simulink model "pseudo_calibrate"  (R2020b)
settings: Solver=VariableStepAuto  StartTime=0.0  StopTime=10  RelTol=1e-3
values from neighbouring files (symbols this model uses):
  B = 0.05    [md.m]    (also in pid.m; pinolo.m)
  J = 0.008    [md.m]    (also in pid.m; pinolo.m)
  KM = 0.22    [md.m]    (also in pid.m; pinolo.m)
  L = 0.0014    [md.m]    (also in pid.m; pinolo.m)
  MAX_SPEED = 330    [md.m]    (also in pid.m; pinolo.m)
  R = 2    [md.m]    (also in pid.m; pinolo.m)
  th = 50    [md.m]    (also in pid.m; pinolo.m)
  tl = 40    [md.m]    (also in pid.m; pinolo.m)
undefined symbols (not defined in the file or in its folder): den, num
libraries: simulink x2
settings Model: Creator=Titania  LastModifiedBy=Titania

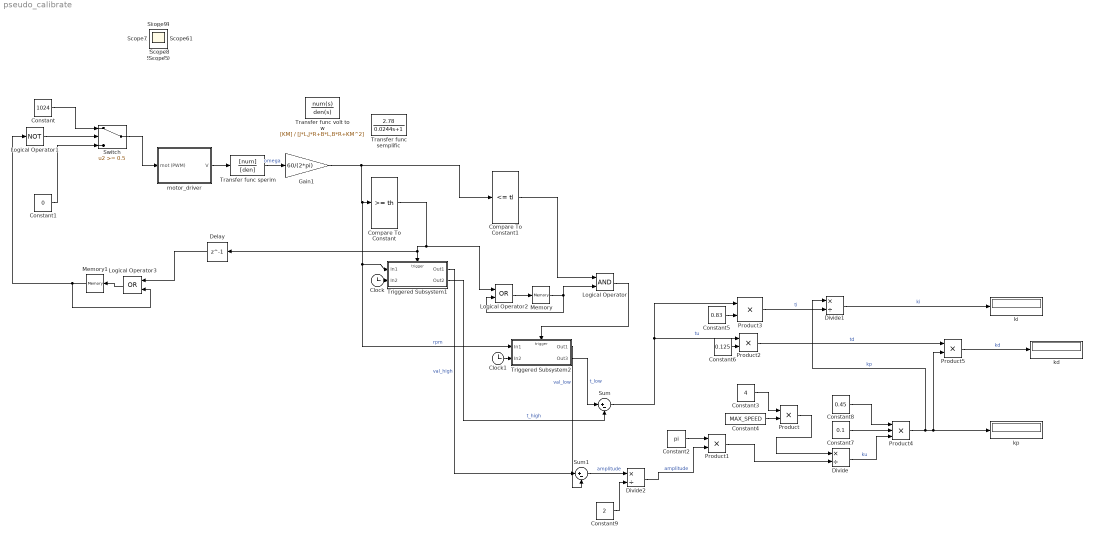
== system pseudo_calibrate ==
  Clock : Clock
  Clock1 : Clock
  Compare To Constant : simulink/Logic and Bit Operations/Compare To Constant  relop=>=  const=th  OutDataTypeStr=boolean
  Compare To Constant1 : simulink/Logic and Bit Operations/Compare To Constant  relop=<=  const=tl  OutDataTypeStr=boolean
  Constant : Constant  Value=1024
  Constant1 : Constant  Value=0
  Constant2 : Constant  Value=pi
  Constant3 : Constant  Value=4
  Constant4 : Constant  Value=MAX_SPEED
  Constant5 : Constant  Value=0.83
  Constant6 : Constant  Value=0.125
  Constant7 : Constant  Value=0.1
  Constant8 : Constant  Value=0.45
  Constant9 : Constant  Value=2
  Delay : Delay  DelayLength=1  InitialCondition=0
  Divide : Product  Inputs=*/
  Divide1 : Product  Inputs=*/
  Divide2 : Product  Inputs=*/
  Gain1 : Gain  Gain=60/(2*pi)
  Logical Operator : Logic  AllPortsSameDT=off  OutDataTypeStr=boolean
  Logical Operator1 : Logic  Operator=NOT  AllPortsSameDT=off  OutDataTypeStr=boolean
  Logical Operator2 : Logic  Operator=OR  AllPortsSameDT=off  OutDataTypeStr=boolean
  Logical Operator3 : Logic  Operator=OR  AllPortsSameDT=off  OutDataTypeStr=boolean
  Memory : Memory
  Memory1 : Memory
  Product{,1..3,5} (5 alike) : Product
  Product4 : Product  Inputs=3  OutDataTypeStr=single
  Sum : Sum  Inputs=|+-
  Sum1 : Sum  Inputs=|+-
  Switch : Switch  Threshold=0.5
  Transfer func semplific : TransferFcn  Numerator=[2.78]  Denominator=[0.0244,1]
  Transfer func sperim : TransferFcn  Numerator=[num]  Denominator=[den]
  Transfer func volt to w : TransferFcn  Numerator=[KM]  Denominator=[J*L,J*R+B*L,B*R+KM^2]
  Triggered Subsystem1 : Subsystem  TreatAsAtomicUnit=on
  Triggered Subsystem2 : Subsystem  TreatAsAtomicUnit=on
  kd : Display
  ki : Display
  kp : Display
  motor_driver : Subsystem
  Scope{,1..11} (12 alike) : Scope
  wires:
  motor_driver/1(V) -> Transfer func sperim/1
  Transfer func sperim/1 -> Gain1/1  "omega"
  Compare To Constant/1 -> Triggered Subsystem1/Trigger, Delay/1, Logical Operator2/1
  Triggered Subsystem1/1(Out1) -> Sum1/1  "val_high"
  Logical Operator/1 -> Triggered Subsystem2/Trigger
  Compare To Constant1/1 -> Logical Operator/1
  Clock/1 -> Triggered Subsystem1/2(In2)
  Triggered Subsystem1/2(Out2) -> Sum/2  "t_high"
  Clock1/1 -> Triggered Subsystem2/2(In2)
  Triggered Subsystem2/1(Out1) -> Sum1/2  "val_low"
  Triggered Subsystem2/2(Out3) -> Sum/1  "t_low"
  Sum/1 -> Product2/1, Product3/1  "tu"
  Divide2/1 -> Product1/2  "amplitude"
  Constant2/1 -> Product1/1
  Constant3/1 -> Product/1
  Constant4/1 -> Product/2
  Product1/1 -> Divide/2
  Product/1 -> Divide/1
  Divide/1 -> Product4/3  "ku"
  Constant5/1 -> Product3/2
  Constant6/1 -> Product2/2
  Product3/1 -> Divide1/2  "ti"
  Product2/1 -> Product5/1  "td"
  Constant7/1 -> Product4/2
  Constant8/1 -> Product4/1
  Product4/1 -> Divide1/1, Product5/2, kp/1  "kp"
  Delay/1 -> Logical Operator3/1
  Switch/1 -> motor_driver/1(mot (PWM))
  Constant/1 -> Switch/1
  Constant1/1 -> Switch/3
  Logical Operator1/1 -> Switch/2
  Logical Operator2/1 -> Memory/1
  Memory/1 -> Logical Operator2/2, Logical Operator/2
  Logical Operator3/1 -> Memory1/1
  Memory1/1 -> Logical Operator1/1, Logical Operator3/2
  Divide1/1 -> ki/1  "ki"
  Product5/1 -> kd/1  "kd"
  Gain1/1 -> Compare To Constant1/1, Triggered Subsystem2/1(In1), Triggered Subsystem1/1(In1), Compare To Constant/1  "rpm"
  Constant9/1 -> Divide2/2
  Sum1/1 -> Divide2/1  "amplitude"

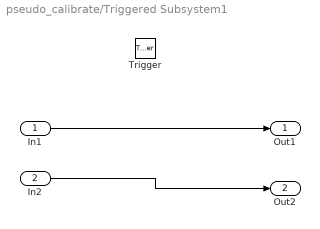
== system pseudo_calibrate/Triggered Subsystem1 ==
  In1 : Inport
  In2 : Inport  Port=2
  Trigger : TriggerPort  VariantControl=Variant
  Out1 : Outport
  Out2 : Outport  Port=2
  wires:
  In1/1 -> Out1/1
  In2/1 -> Out2/1

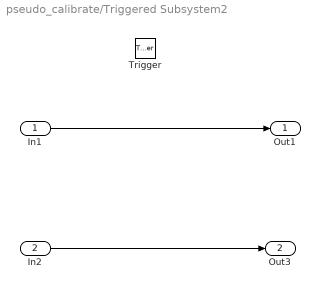
== system pseudo_calibrate/Triggered Subsystem2 ==
  In1 : Inport
  In2 : Inport  Port=2
  Trigger : TriggerPort  VariantControl=Variant
  Out1 : Outport
  Out3 : Outport  Port=2
  wires:
  In1/1 -> Out1/1
  In2/1 -> Out3/1

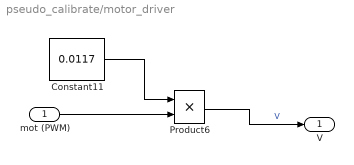
== system pseudo_calibrate/motor_driver ==
  mot (PWM) : Inport
  Constant11 : Constant  Value=0.0117
  Product6 : Product
  V : Outport
  wires:
  Constant11/1 -> Product6/1
  Product6/1 -> V/1  "V"
  mot (PWM)/1 -> Product6/2
